simulink model "non_ss_kalmf_Observer"  (R2022b)
settings: Solver=VariableStepAuto  StartTime=0.0  StopTime=10.0  RelTol=1e-3
settings Model: Creator=hp_desktop  LastModifiedBy=hp_desktop
settings DataIOCC: SaveOutput=off  SaveTime=off

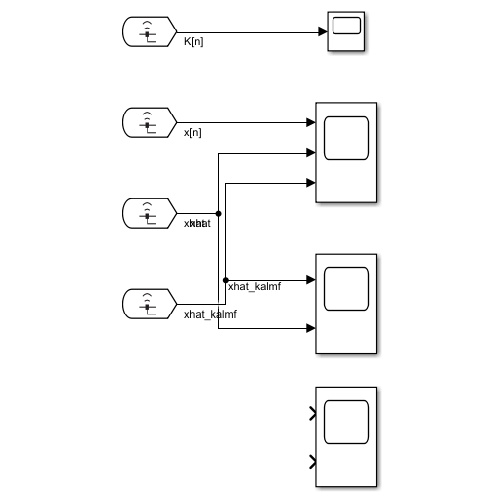
[thumbnail: Simulink's stored preview of the top-level diagram]
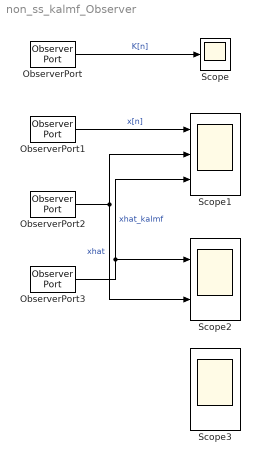
== system non_ss_kalmf_Observer ==
  ObserverPort{,1..3} (4 alike) : ObserverPort
  Scope : Scope
  Scope1 : Scope  NumInputPorts=3
  Scope2 : Scope  NumInputPorts=2
  Scope3 : Scope  NumInputPorts=2
  wires:
  ObserverPort/1 -> Scope/1  "K[n]"
  ObserverPort1/1 -> Scope1/1  "x[n]"
  ObserverPort2/1 -> Scope2/2, Scope1/2  "xhat"
  ObserverPort3/1 -> Scope1/3, Scope2/1  "xhat_kalmf"
